simulink model "stateSpaceModel"  (R2020b)
settings: Solver=VariableStepAuto  StartTime=0.0  StopTime=10.0  RelTol=1e-3
settings Model: Creator=kuzub  LastModifiedBy=kuzub

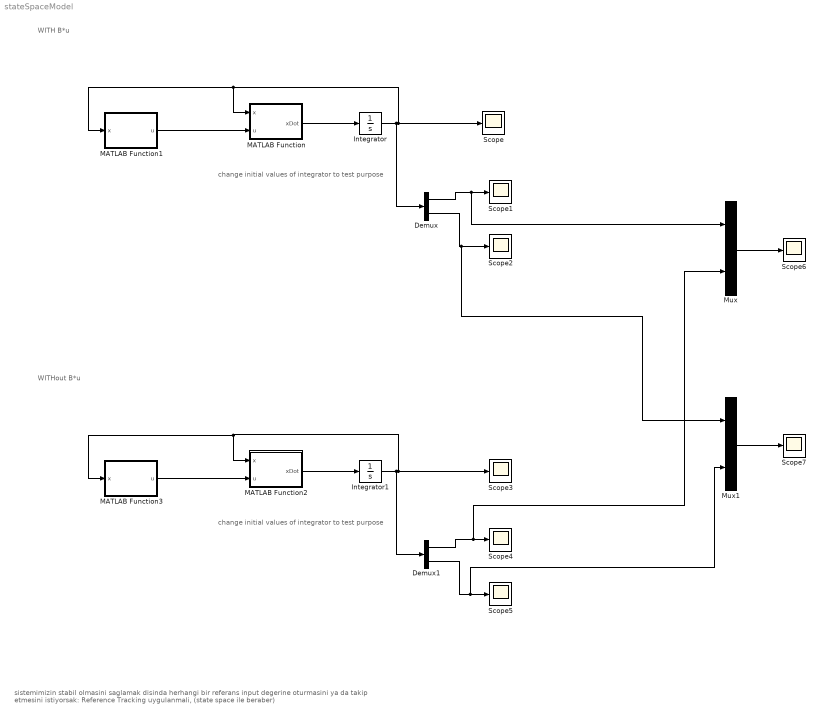
== system stateSpaceModel ==
  note: sistemimizin stabil olmasini saglamak disinda herhangi bir referans input degerine oturmasini ya da takip etmesini istiyorsak:
      | 	Reference Tracking uygulanmali, (state space ile beraber)
  note: WITH B*u
  note: change initial values of integrator to test purpose
  note: WITHout B*u
  note: change initial values of integrator to test purpose
  Demux : Demux  Outputs=2
  Demux1 : Demux  Outputs=2
  Integrator : Integrator  InitialCondition=[100;20]
  Integrator1 : Integrator  InitialCondition=[100;20]
  MATLAB Function : MATLAB Function  TreatAsAtomicUnit=on
  MATLAB Function1 : MATLAB Function  TreatAsAtomicUnit=on
  MATLAB Function2 : MATLAB Function  TreatAsAtomicUnit=on
  MATLAB Function3 : MATLAB Function  TreatAsAtomicUnit=on
  Mux : Mux  Inputs=2
  Mux1 : Mux  Inputs=2
  Scope{,1..7} (8 alike) : Scope
  wires:
  MATLAB Function/1(xDot) -> Integrator/1
  Integrator/1 -> Scope/1, MATLAB Function1/1(x), MATLAB Function/1(x), Demux/1
  MATLAB Function1/1(u) -> MATLAB Function/2(u)
  Demux/1 -> Mux/1, Scope1/1
  Demux/2 -> Mux1/1, Scope2/1
  Demux1/2 -> Mux1/2, Scope5/1
  Demux1/1 -> Mux/2, Scope4/1
  MATLAB Function3/1(u) -> MATLAB Function2/2(u)
  Integrator1/1 -> Demux1/1, MATLAB Function2/1(x), MATLAB Function3/1(x), Scope3/1
  MATLAB Function2/1(xDot) -> Integrator1/1
  Mux/1 -> Scope6/1
  Mux1/1 -> Scope7/1

== matlab function stateSpaceModel/MATLAB Function ==
  data: x input; u input; xDot output
function xDot = fcn(x, u)
    %
    % System Constants
    R = 0.55;
    J = 0.09;
    Kt = 85*10^-3;
    L = 25*10^-3;
    b = 0.05;
    %
    %% State Space Matrix
    %
    a00 = -R/L;
    a01 = -Kt/L;
    a10 = Kt/J;
    a11 = -b/J;
    %
    b00 = 1/L;
    b10 = 0;
    %
    A = [a00, a01;
         a10, a11];
    % 
    B = [b00; b10];
    %
    xDot = A*x + Bu;
end

== matlab function stateSpaceModel/MATLAB Function2 ==
  data: x input; u input; xDot output
function xDot = fcn(x, u)
    %
    % System Constants
    R = 0.55;
    J = 0.09;
    Kt = 85*10^-3;
    L = 25*10^-3;
    b = 0.05;
    %
    %% State Space Matrix
    %
    a00 = -R/L;
    a01 = -Kt/L;
    a10 = Kt/J;
    a11 = -b/J;
    %
    b00 = 1/L;
    b10 = 0;
    %
    A = [a00, a01;
         a10, a11];
    % 
    B = [b00; b10];
    %
    xDot = A*x;
end

== matlab function stateSpaceModel/MATLAB Function3 ==
  data: x input; u output
function u = fcn(x)
%
%Calculated K matrix
K = [ -0.3389    0.3202];
%
u = -K*x;
%
end

== matlab function stateSpaceModel/MATLAB Function1 ==
  data: x input; u output
function u = fcn(x)
%
%Calculated K matrix
K = [ -0.3389    0.3202];
%
u = -K*x;
%
end
